simulink model "CommutationSimv2"  (Simulink 7.8)
settings: Solver=FixedStepDiscrete  StartTime=0.0  StopTime=1  FixedStep=.00001  RelTol=1e-3
undefined symbols (not defined in the file): abc, alphabeta, DiscIntNeverNeededParam, dq, MicrochipMotorControlTools, to
libraries: powerlib x9, simulink x7
settings Model: Creator=Marx  LastModifiedBy=Pavlo
settings DataIOCC: LimitDataPoints=off

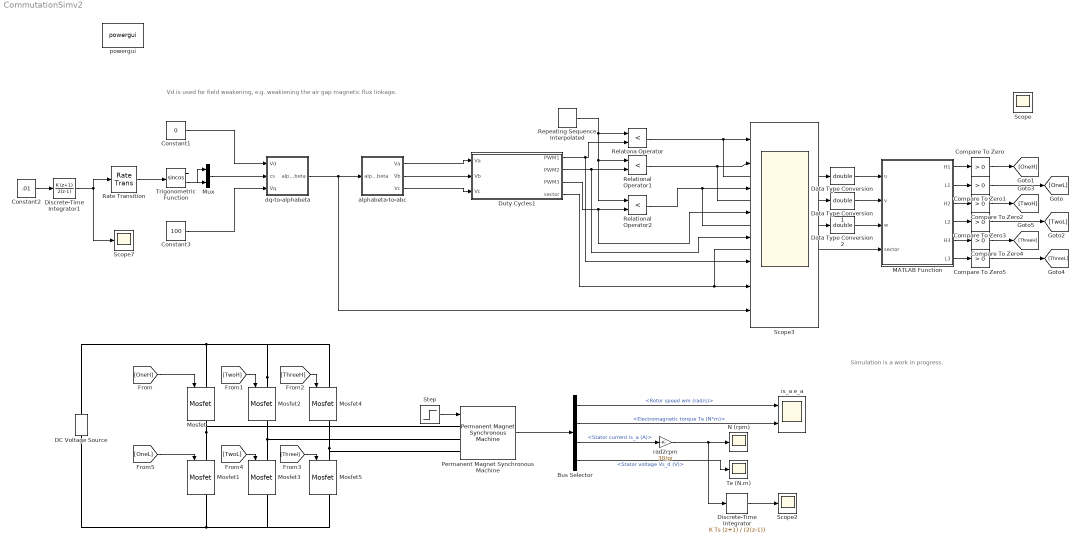
== system CommutationSimv2 ==
  note: Vd is used for field weakening, e.g. weakiening the air gap magnetic flux linkage.
  note: Simulation is a work in progress.
  Bus Selector : BusSelector  OutputSignals=Rotor speed wm (rad/s),Electromagnetic torque Te (N*m),Stator current is_a (A),Stator voltage Vs_d (V)
  Compare To Zero{,1..5} (6 alike) : simulink/Logic and Bit Operations/Compare To Zero  relop=>  OutDataTypeStr=boolean
  Constant1 : Constant  Value=0
  Constant2 : Constant  Value=.01
  Constant3 : Constant  Value=100
  DC Voltage Source : powerlib/Electrical Sources/DC Voltage Source  Amplitude=48  Measurements=None
  Data Type Conversion : DataTypeConversion  OutDataTypeStr=double
  Data Type Conversion1 : DataTypeConversion  OutDataTypeStr=double
  Data Type Conversion2 : DataTypeConversion  OutDataTypeStr=double
  Discrete-Time Integrator : DiscreteIntegrator  IntegratorMethod=Integration: Trapezoidal  SampleTime=.00001  ICPrevOutput=DiscIntNeverNeededParam  ICPrevScaledInput=DiscIntNeverNeededParam
  Discrete-Time Integrator1 : DiscreteIntegrator  IntegratorMethod=Accumulation: Trapezoidal  SampleTime=.0001  ICPrevOutput=DiscIntNeverNeededParam  ICPrevScaledInput=DiscIntNeverNeededParam
  Duty Cycles1 : MATLAB Function  TreatAsAtomicUnit=on
  MATLAB Function : MATLAB Function  TreatAsAtomicUnit=on
  Mosfet{,1..5} (6 alike) : powerlib/Power Electronics/Mosfet  Ron=0.1  Lon=0  Rd=0.01  Vfd=0  IC=0  Rs=1e5  Cs=inf  Measurements=on
  Mux : Mux  Inputs=2
  N (rpm) : Scope
      settings: TimeRange=0.2  YMin=-37.5  YMax=17.5  SaveName=N
  Permanent Magnet Synchronous Machine : powerlib/Machines/Permanent Magnet Synchronous Machine  NbPhases=3  FluxDistribution=Sinusoidal  RotorType=Round  MechanicalLoad=Torque Tm  PresetModel=No  ShowDetailedParameters=on  Resistance=4.82  Inductance=8.5e-3  dqInductances=[8.5e-3,8.5e-3]  La=0.000835  MachineConstant=Flux linkage established by magnets (V.s)  Flux=0.07145  VoltageCst=51.8384  TorqueCst=0.4287  Flat=120  Mechanical=[0.00062 0.0003035 4 0]  PolePairs=4  InitialConditions=[0,0, 0,0]  InitialConditions5ph=[0 0 0 0 0 0]  TsPowergui=0  TsBlock=-1  RefAngle=90 degrees behind phase A axis (modified Park)
  Rate Transition : RateTransition  OutPortSampleTime=.00001
  Relational Operator1 : RelationalOperator  Operator=<  OutDataTypeStr=boolean
  Relational Operator2 : RelationalOperator  Operator=<  OutDataTypeStr=boolean
  Relatona Operator : RelationalOperator  Operator=<  OutDataTypeStr=boolean
  Repeating Sequence Interpolated : simulink/Sources/Repeating Sequence Interpolated  OutValues=[0 10000].'  TimeValues=[0 .001].'  LookUpMeth=Interpolation-Use End Values  tsamp=.00001  OutMin=[]  OutMax=[]  OutDataTypeStr=double  OutputDataTypeScalingMode=double  OutDataType=fixdt(0,8)  OutScaling=2^-10
  Scope : Scope
  Scope2 : Scope
      settings: YMin=-2.25  YMax=2.75  SaveName=ScopeData7  MaxDataPoints=50000
  Scope3 : Scope  NumInputPorts=8
      settings: YMin=-0.2~-0.2~-0.2~-20~-20~-20~-1~-100  YMax=1.2~1.2~1.2~10020~10020~10020~8~100  MaxDataPoints=500000
  Scope7 : Scope
      settings: YMin=0  YMax=9500  SaveName=ScopeData8
  Step : Step  SampleTime=.00001
  Te (N.m) : Scope
      settings: TimeRange=1  YMin=-35  YMax=35  SaveName=N1
  Trigonometric Function : Trigonometry  Operator=sincos
  alphabeta-to-abc : Subsystem  AncestorBlock=MicrochipMotorControlTools/alphabeta-to-abc
  dq-to-alphabeta : Subsystem  AncestorBlock=MicrochipMotorControlTools/dq-to-alphabeta
  is_a e_a : Scope  NumInputPorts=2
      settings: TimeRange=0.2  YMin=-32.5~-0.75  YMax=2.5~3.5  SaveName=IE
  powergui : powerlib/powergui  Priority=1  SimulationMode=Discrete  SolverType=Tustin  SampleTime=.00001  frequency=60  SPID=off  DisableSnubberDevices=off  DisableRonSwitches=off  DisableVfSwitches=off  SwTol=0  Interpol=off  DisplayEquations=off  FunctionMessages=off  frequencyindice=0  Pbase=100e6  ErrMax=1e-4  Iterations=50  UnitsV=kV  UnitsW=MW  echomessages=off  HookPort=off  EnableUseOfTLC=off  x0status=blocks  RestoreLinks=warning  ResistiveCurrentMeasurement=off  Ylog=off  Xlog=on  ShowGrid=off  save=off  variable=ZData  ZoomFFT=off  StartTime=0.0  cycles=1  DisplayStyle=1  FreqAxis=off  MaxFrequency=1000  frequencyindicesteady=1  display=off  methode=off
  rad2rpm : Gain  Gain=30/pi
  wires:
  Step/1 -> Permanent Magnet Synchronous Machine/1
  [OneH] -> Mosfet/1
  [TwoH] -> Mosfet2/1
  [ThreeH] -> Mosfet4/1
  [Threel] -> Mosfet5/1
  [TwoL] -> Mosfet3/1
  [OneL] -> Mosfet1/1
  rad2rpm/1 -> N (rpm)/1, Discrete-Time Integrator/1
  Bus Selector/1 -> is_a e_a/1  "<Rotor speed wm (rad/s)>"
  Permanent Magnet Synchronous Machine/1 -> Bus Selector/1
  Bus Selector/2 -> is_a e_a/2  "<Electromagnetic torque Te (N*m)>"
  Bus Selector/3 -> rad2rpm/1  "<Stator current is_a (A)>"
  Bus Selector/4 -> Te (N.m)/1  "<Stator voltage Vs_d (V)>"
  Discrete-Time Integrator/1 -> Scope2/1
  Discrete-Time Integrator1/1 -> Scope7/1, Rate Transition/1
  Constant2/1 -> Discrete-Time Integrator1/1
  Mux/1 -> dq-to-alphabeta/2(cs)
  dq-to-alphabeta/1(alphabeta) -> alphabeta-to-abc/1(alphabeta), Scope3/8
  alphabeta-to-abc/1(Va) -> Duty Cycles1/1(Va)
  alphabeta-to-abc/2(Vb) -> Duty Cycles1/2(Vb)
  alphabeta-to-abc/3(Vc) -> Duty Cycles1/3(Vc)
  Constant1/1 -> dq-to-alphabeta/1(Vd)
  Constant3/1 -> dq-to-alphabeta/3(Vq)
  Trigonometric Function/2 -> Mux/1
  Trigonometric Function/1 -> Mux/2
  Duty Cycles1/1(PWM1) -> Relatona Operator/2, Scope3/6
  Duty Cycles1/2(PWM2) -> Relational Operator1/2, Scope3/5
  Duty Cycles1/3(PWM3) -> Relational Operator2/2, Scope3/4
  Repeating Sequence Interpolated/1 -> Relatona Operator/1, Relational Operator2/1, Relational Operator1/1
  Rate Transition/1 -> Trigonometric Function/1
  Relatona Operator/1 -> Data Type Conversion/1, Scope3/1
  Relational Operator1/1 -> Data Type Conversion1/1, Scope3/2
  Relational Operator2/1 -> Data Type Conversion2/1, Scope3/3
  Duty Cycles1/4(sector) -> MATLAB Function/4(sector), Scope3/7
  MATLAB Function/1(H1) -> Compare To Zero/1
  MATLAB Function/2(L1) -> Compare To Zero1/1
  MATLAB Function/3(H2) -> Compare To Zero2/1
  MATLAB Function/4(L2) -> Compare To Zero3/1
  MATLAB Function/5(H3) -> Compare To Zero4/1
  MATLAB Function/6(L3) -> Compare To Zero5/1
  Compare To Zero/1 -> [OneH]
  Compare To Zero1/1 -> [OneL]
  Compare To Zero2/1 -> [TwoH]
  Compare To Zero3/1 -> [TwoL]
  Compare To Zero4/1 -> [ThreeH]
  Compare To Zero5/1 -> [ThreeL]
  Data Type Conversion1/1 -> MATLAB Function/2(v)
  Data Type Conversion/1 -> MATLAB Function/1(u)
  Data Type Conversion2/1 -> MATLAB Function/3(w)
  connections:
  DC Voltage Source/RConn1 -- Mosfet4/LConn1 -- Mosfet2/LConn1 -- Mosfet/LConn1
  Mosfet/RConn1 -- Mosfet1/LConn1 -- Permanent Magnet Synchronous Machine/LConn1
  Mosfet2/RConn1 -- Mosfet3/LConn1 -- Permanent Magnet Synchronous Machine/LConn2
  Mosfet4/RConn1 -- Mosfet5/LConn1 -- Permanent Magnet Synchronous Machine/LConn3
  Mosfet5/RConn1 -- Mosfet3/RConn1 -- DC Voltage Source/LConn1 -- Mosfet1/RConn1

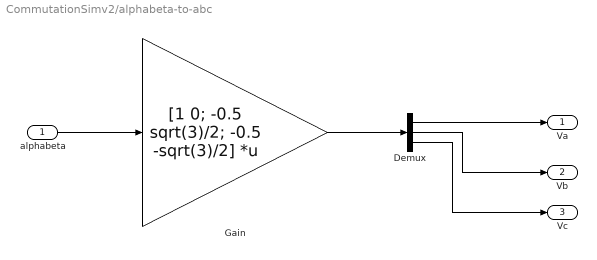
== system CommutationSimv2/alphabeta-to-abc ==
  alphabeta : Inport
  Demux : Demux  Outputs=3
  Gain : Gain  Gain=[1 0; -0.5 sqrt(3)/2; -0.5 -sqrt(3)/2]  Multiplication=Matrix(K*u)  OutDataTypeStr=single
  Va : Outport  OutDataTypeStr=single
  Vb : Outport  Port=2  OutDataTypeStr=single
  Vc : Outport  Port=3  OutDataTypeStr=single
  wires:
  alphabeta/1 -> Gain/1
  Gain/1 -> Demux/1
  Demux/1 -> Va/1
  Demux/2 -> Vb/1
  Demux/3 -> Vc/1

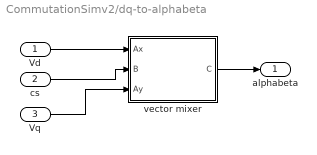
== system CommutationSimv2/dq-to-alphabeta ==
  Vd : Inport
  cs : Inport  Port=2
  Vq : Inport  Port=3
  vector mixer : Subsystem  AncestorBlock=MicrochipMotorControlTools/vector mixer
  alphabeta : Outport
  wires:
  cs/1 -> vector mixer/2(B)
  Vd/1 -> vector mixer/1(Ax)
  vector mixer/1(C) -> alphabeta/1
  Vq/1 -> vector mixer/3(Ay)

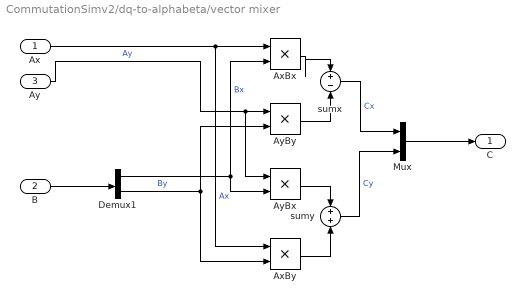
== system CommutationSimv2/dq-to-alphabeta/vector mixer ==
  Ax : Inport
  B : Inport  Port=2
  Ay : Inport  Port=3
  AxBx : Product  RndMeth=Zero  OutDataTypeStr=Inherit: Same as first input
  AxBy : Product  RndMeth=Zero  OutDataTypeStr=Inherit: Same as first input
  AyBx : Product  RndMeth=Zero  OutDataTypeStr=Inherit: Same as first input
  AyBy : Product  RndMeth=Zero  OutDataTypeStr=Inherit: Same as first input
  Demux1 : Demux  Outputs=2
  Mux : Mux  Inputs=2
  sumx : Sum  Inputs=+|-
  sumy : Sum  Inputs=+|+
  C : Outport
  wires:
  sumx/1 -> Mux/1  "Cx"
  B/1 -> Demux1/1
  Demux1/1 -> AyBx/2, AxBx/2  "Bx"
  Demux1/2 -> AxBy/2, AyBy/2  "By"
  sumy/1 -> Mux/2  "Cy"
  AxBy/1 -> sumy/2
  AyBx/1 -> sumy/1
  AxBx/1 -> sumx/1
  AyBy/1 -> sumx/2
  Ay/1 -> AyBy/1, AyBx/1  "Ay"
  Ax/1 -> AxBy/1, AxBx/1  "Ax"
  Mux/1 -> C/1

== matlab function MATLAB Function ==
  data: u input double; H1 output double; v input double; w input double; sector input double; L1 output double; H2 output double; L2 output boolean; H3 output boolean; L3 output boolean
function [H1, L1, H2, L2, H3, L3] = fcn(u, v, w, sector)
%#codegen

    if (sector == 3)
        H1 = u;
        H2 = 0;
        H3 = 0;
        L1 = 0;
        L2 = u;
        L3 = u;
    elseif (sector == 1)
        H1 = u;
        H2 = v;
        H3 = 0;
        L1 = 0;
        L2 = 0;
        L3 = 1;
    elseif (sector == 5)
        H1 = 0;
        H2 = v;
        H3 = 0;
        L1 = v;
        L2 = 0;
        L3 = v;
    elseif (sector == 4)
        H1 = 0;
        H2 = v;
        H3 = w;
        L1 = 1;
        L2 = 0;
        L3 = 0;
    elseif (sector == 6)
        H1 = 0;
        H2 = 0;
        H3 = w;
        L1 = w;
        L2 = w;
        L3 = 0;
    else
        H1 = u;
        H2 = 0;
        H3 = w;
        L1 = 0;
        L2 = 1;
        L3 = 0;
    end
end

== matlab function Duty Cycles1 ==
  data: PWM1 output single; Va input single; PWM2 output single; PWM3 output single; sector output double; Vb input double; Vc input double
function [PWM1, PWM2, PWM3, sector]  = DutyCycleCalc(Va, Vb, Vc)
%#codegen
PWM = single(100);

Ta = single(0);

if (Va >= 0)
    if (Vb >= 0)
        %Sector 3, 0 - 60 Degrees
        T1 = Vb;
        T2 = Va;
    
        T1 = T1*PWM;
        T2 = T2*PWM;
        Tc = (PWM-T1-T2)/2;
        Tb = Ta + T1;
        Ta = Tb + T2;
    
        PWM1 = single(0);
        PWM2 = Tb;
        PWM3 = Ta;
        sector = single(3);
    else
        if (Vc >= 0)
           %Sector 5, 120 - 180 Degrees
            T1 = Va;
            T2 = Vc;
    
            T1 = T1*PWM;
            T2 = T2*PWM;
            Tc = (PWM-T1-T2)/2;
            Tb = Ta + T1;
            Ta = Tb + T2;
    
            PWM1 = Ta;
            PWM2 = single(0);
            PWM3 = Tb;
            sector = single(5);
        else
            %Sector 1, 60 - 120 Degrees
            T1 = -Vb;
            T2 = -Vc;
    
            T1 = T1*PWM;
            T2 = T2*PWM;
            Tc = (PWM-T1-T2)/2;
            Tb = Ta + T1;
            Ta = Tb + T2;
    
            PWM1 = Tb;
            PWM2 = single(0);
            PWM3 = Ta;
            sector = single(1);
        end
    end
else
    if (Vb >= 0)
        if (Vc >= 0)
            %Sector 6, 240 - 300 Degrees
            T1 = Vc;
            T2 = Vb;
    
            T1 = T1*PWM;
            T2 = T2*PWM;
            Tc = (PWM-T1-T2)/2;
            Tb = Ta + T1;
            Ta = Tb + T2;
    
            PWM1 = Tb;
            PWM2 = Ta;
            PWM3 = single(0);
            sector = single(6);
        else
            %Sector 2, 300 - 0 Degrees
            T1 = -Vc;
            T2 = -Va;
    
            T1 = T1*PWM;
            T2 = T2*PWM;
            Tc = (PWM-T1-T2)/2;
            Tb = Ta + T1;
            Ta = Tb + T2;
    
            PWM1 = single(0);
            PWM2 = Ta;
            PWM3 = Tb;
            sector = single(2);
        end
    else
        %Sector 4, 180 - 240 Degrees
        T1 = -Va;
        T2 = -Vb;
    
        T1 = T1*PWM;
        T2 = T2*PWM;
        Tc = (PWM-T1-T2)/2;
        Tb = Ta + T1;
        Ta = Tb + T2;
    
        PWM1 = Ta;
        PWM2 = Tb;
        PWM3 = single(0);
        sector = single(4);
    end
end

end
